simulink model "input_state_lin"  (R2025a)
settings: Solver=VariableStepAuto  StartTime=0.0  StopTime=10  MaxStep=1e-3  RelTol=1e-3
values from neighbouring files (symbols this model uses):
  a = 1    [input_state_lin_param.m]
  x1_0 = 0    [input_state_lin_param.m]
  x2_0 = 0    [input_state_lin_param.m]
libraries: slpidlib x1
settings Model: Creator=amoralesma  LastModifiedBy=amoralesma

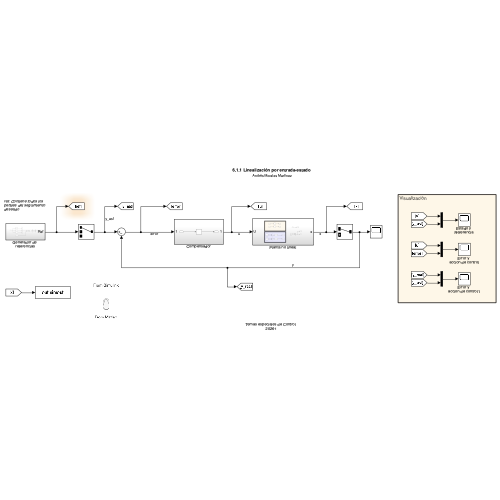
[thumbnail: Simulink's stored preview of the top-level diagram]
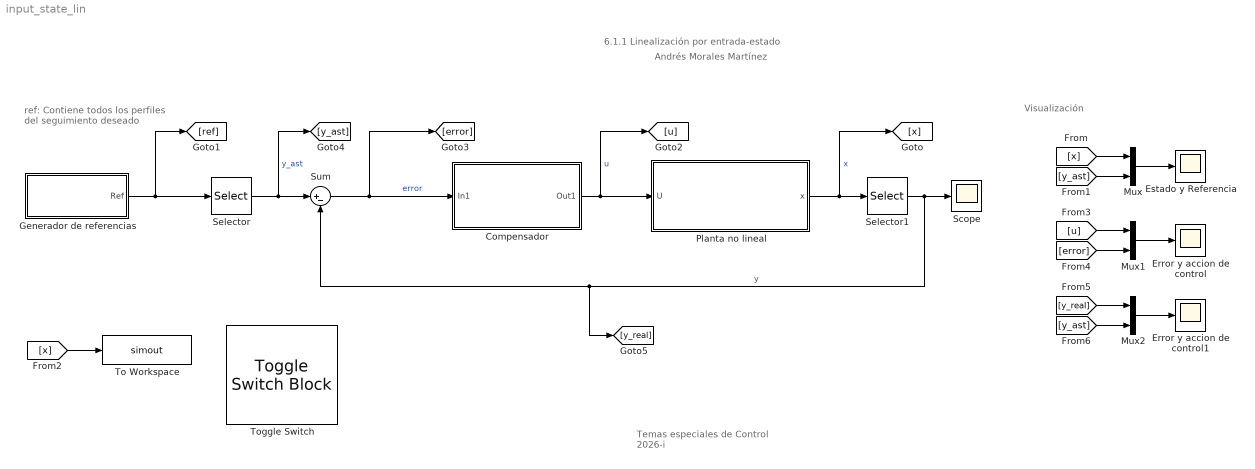
== system input_state_lin ==
  note: ref: Contiene todos los
      | perfiles del seguimiento
      | deseado
  note: Visualización
  note: Temas especiales de Control
      | 2026-i
  note: 6.1.1 Linealización por entrada-estado
  note: Andrés Morales Martínez
  Compensador : Subsystem
  Error y accion de control : Scope
      settings: ActiveDisplayYMinimum=-2.336578750988239  ActiveDisplayYMaximum=2.5265986773116764  DataLoggingVariableName=ScopeData2
  Error y accion de control1 : Scope
      settings: ActiveDisplayYMinimum=-1.2499999148694403  ActiveDisplayYMaximum=1.2499999903536541  DataLoggingVariableName=ScopeData4
  Estado y Referencia : Scope
      settings: ActiveDisplayYMinimum=-1.3860022469354711  ActiveDisplayYMaximum=1.460127424016846
  Generador de referencias : Subsystem
  Mux : Mux  Inputs=2
  Mux1 : Mux  Inputs=2
  Mux2 : Mux  Inputs=2
  Planta no lineal : Subsystem
  Scope : Scope
      settings: ActiveDisplayYMinimum=-1  ActiveDisplayYMaximum=1
  Selector : Selector  InputPortWidth=3  IndexOptions=Index vector (dialog)  Indices=[1]  OutputSizes=1
  Selector1 : Selector  InputPortWidth=2  IndexOptions=Index vector (dialog)  Indices=[1]  OutputSizes=1
  Sum : Sum  Inputs=|+-
  To Workspace : ToWorkspace  VariableName=simout  SaveFormat=Timeseries  SampleTime=-1
  Toggle Switch : ToggleSwitchBlock  LabelPosition=Hide
  wires:
  Planta no lineal/1(x) -> Selector1/1, [x]  "x"
  [x] -> Mux/1
  Mux/1 -> Estado y Referencia/1
  [y_ast] -> Mux/2
  Compensador/1(Out1) -> [u], Planta no lineal/1(U)  "u"
  [x] -> To Workspace/1
  Sum/1 -> [error], Compensador/1(In1)  "error"
  [u] -> Mux1/1
  [error] -> Mux1/2
  Mux1/1 -> Error y accion de control/1
  Generador de referencias/1(Ref) -> Selector/1, [ref]
  Selector/1 -> Sum/1, [y_ast]  "y_ast"
  Selector1/1 -> [y_real], Sum/2, Scope/1  "y"
  [y_real] -> Mux2/1
  [y_ast] -> Mux2/2
  Mux2/1 -> Error y accion de control1/1

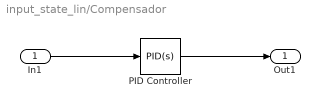
== system input_state_lin/Compensador ==
  In1 : Inport
  PID Controller : slpidlib/PID Controller  Controller=PID  Form=Parallel  TimeDomain=Continuous-time  UseExternalTs=off  SampleTime=-1  IntegratorMethod=Forward Euler  FilterMethod=Forward Euler  ControllerParametersSource=internal  P=1  I=1  UseKiTs=off  D=0  UseExternalDerivativeSource=off  N=100  UseFilter=on  TunerSelectOption=Transfer Function Based (PID Tuner App)  InitialConditionSource=internal  InitialConditionForIntegrator=0  InitialConditionForFilter=0  DifferentiatorICPrevScaledInput=0  ExternalReset=none  TrackingMode=off  Kt=1  LimitOutput=off  SatLimitsSource=internal  UpperSaturationLimit=inf  LowerSaturationLimit=-inf  LinearizeAsGain=on  AntiWindupMode=none  Kb=1  LimitIntegrator=off  UpperIntegratorSaturationLimit=inf  LowerIntegratorSaturationLimit=-inf  POutMin=[]  POutMax=[]  IOutMin=[]  IOutMax=[]  DOutMin=[]  DOutMax=[]  NOutMin=[]  NOutMax=[]  SumOutMin=[]  SumOutMax=[]  SaturationOutMin=[]  SaturationOutMax=[]  PParamMin=[]  PParamMax=[]  IParamMin=[]  IParamMax=[]  DParamMin=[]  DParamMax=[]  NParamMin=[]  NParamMax=[]  KbParamMin=[]  KbParamMax=[]  KtParamMin=[]  KtParamMax=[]  KbOutMin=[]  KbOutMax=[]  KtOutMin=[]  KtOutMax=[]  IntegratorOutMin=[]  IntegratorOutMax=[]  FilterOutMin=[]  FilterOutMax=[]  SumI1OutMin=[]  SumI1OutMax=[]  SumI2OutMin=[]  SumI2OutMax=[]  SumI3OutMin=[]  SumI3OutMax=[]  SumI4OutMin=[]  SumI4OutMax=[]  SumDOutMin=[]  SumDOutMax=[]  DifferentiatorOutMin=[]  DifferentiatorOutMax=[]  FilterDiffOutCoefMin=[]  FilterDiffOutCoefMax=[]  ReciprocalOutMin=[]  ReciprocalOutMax=[]  SumDenOutMin=[]  SumDenOutMax=[]  SumNumOutMin=[]  SumNumOutMax=[]  DivideOutMin=[]  DivideOutMax=[]  UdiffTsProdOutMin=[]  UdiffTsProdOutMax=[]  NTsProdOutMin=[]  NTsProdOutMax=[]  UintegralTsProdOutMin=[]  UintegralTsProdOutMax=[]  UngainTsProdOutMin=[]  UngainTsProdOutMax=[]  ClampingZeroOutDataTypeStr=Inherit: Inherit via back propagation  ClampingZeroOutMin=[]  ClampingZeroOutMax=[]  FilterDenConstantOutDataTypeStr=Inherit: Inherit via back propagation  FilterDenConstantOutMin=[]  FilterDenConstantOutMax=[]  PCopyOutDataTypeStr=Inherit: Inherit via back propagation  PCopyOutMin=[]  PCopyOutMax=[]  NCopyOutDataTypeStr=Inherit: Inherit via back propagation  NCopyOutMin=[]  NCopyOutMax=[]  IntegratorContinuousStateAttributes=''  IntegratorStateMustResolveToSignalObject=off  IntegratorRTWStateStorageClass=Auto  FilterContinuousStateAttributes=''  FilterStateMustResolveToSignalObject=off  FilterRTWStateStorageClass=Auto  ParallelPVariant=InternalParameters  IdealPVariant=Disabled  IVariant=InternalParameters  DVariant=InternalParameters  IntegratorVariant=Continuous  SatVariant=Disabled  AWVariant=Passthrough  PCopyVariant=Disabled  TRVariant=Disabled  FdbkBlocksVariant=Forward  IdealPFdbkVariant=Disabled  SatFdbkVariant=Disabled  DerivativeFilterVariant=ContFilter  NVariant=InternalParameters  NCopyVariant=Disabled  FilterICVariant=InternalICsFilter  IntegratorICVariant=InternalICs  ExternalResetVariant=Disabled  TRSumVariant=Passthrough  SumFdbkVariant=Disabled  SumVariant=Sum_PID  TsampFilterVariant=InternalTs  TsampNgainVariant=Passthrough  TsampIntegralVariant=Disabled_SignalSpec  ExternalSaturationOutDataTypeStr=Inherit: Same as second input  DerivativeSourceVariant=ErrorSignal  PreIntVariant=InternalPreInt
  Out1 : Outport
  wires:
  In1/1 -> PID Controller/1
  PID Controller/1 -> Out1/1

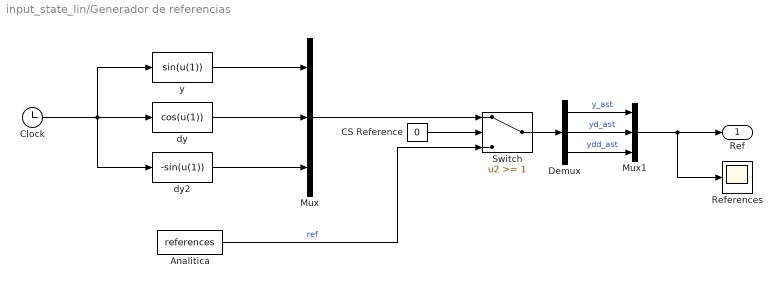
== system input_state_lin/Generador de referencias ==
  Analitica : FromWorkspace  VariableName=references
  CS Reference : Constant  Value=0
  Clock : Clock
  Demux : Demux  Outputs=3
  Mux : Mux  Inputs=3
  Mux1 : Mux  Inputs=3
  References : Scope
      settings: ActiveDisplayYMinimum=-8.9602274514512477  ActiveDisplayYMaximum=8.624403719070644  DataLoggingVariableName=ScopeData3
  Switch : Switch  Threshold=1  SaturateOnIntegerOverflow=off  InputSameDT=off
  dy : Fcn  Expr=cos(u(1))
  dy2 : Fcn  Expr=-sin(u(1))
  y : Fcn  Expr=sin(u(1))
  Ref : Outport
  wires:
  Clock/1 -> dy2/1, dy/1, y/1
  dy2/1 -> Mux/3
  dy/1 -> Mux/2
  y/1 -> Mux/1
  Mux/1 -> Switch/1
  CS Reference/1 -> Switch/2
  Analitica/1 -> Switch/3  "ref"
  Demux/3 -> Mux1/3  "ydd_ast"
  Demux/1 -> Mux1/1  "y_ast"
  Demux/2 -> Mux1/2  "yd_ast"
  Switch/1 -> Demux/1
  Mux1/1 -> References/1, Ref/1

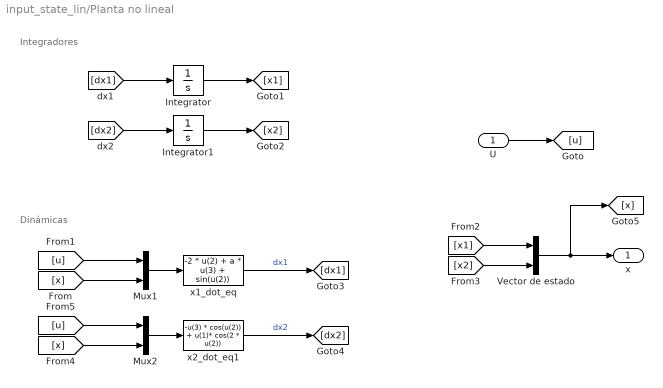
== system input_state_lin/Planta no lineal ==
  note: Integradores
  note: Dinámicas
  U : Inport
  Integrator : Integrator  InitialCondition=x1_0
  Integrator1 : Integrator  InitialCondition=x2_0
  Mux1 : Mux  Inputs=2
  Mux2 : Mux  Inputs=2
  Vector de estado : Mux  Inputs=2
  x1_dot_eq : Fcn  Expr=-2 * u(2) + a * u(3) + sin(u(2))
  x2_dot_eq1 : Fcn  Expr=-u(3) * cos(u(2)) + u(1)* cos(2 * u(2))
  x : Outport
  wires:
  U/1 -> [u]
  [dx1] -> Integrator/1
  [dx2] -> Integrator1/1
  Integrator/1 -> [x1]
  Integrator1/1 -> [x2]
  [x1] -> Vector de estado/1
  [x2] -> Vector de estado/2
  Vector de estado/1 -> [x], x/1
  Mux1/1 -> x1_dot_eq/1
  [u] -> Mux1/1
  [x] -> Mux1/2
  x1_dot_eq/1 -> [dx1]  "dx1"
  [u] -> Mux2/1
  Mux2/1 -> x2_dot_eq1/1
  [x] -> Mux2/2
  x2_dot_eq1/1 -> [dx2]  "dx2"
